simulink model "missile_model"  (R2025a)
settings: Solver=ode4  StartTime=0.0  StopTime=40  FixedStep=0.01  RelTol=1e-5
PreLoadFcn:
  | [aircraft, state] = astDehavillandBeaver();
  | thrustX = getCoefficient(aircraft,"CX","Propeller",Component="Propeller");
model workspace (MATLAB code in the model file + MAT data in the model file):
  inputs0.time = 0
  inputs0.signals(1).dimensions = 1
  inputs0.signals(1).values = -0.104711430294
  inputs0.signals(2).dimensions = 1
  inputs0.signals(2).values = -0.0698725229544
  inputs0.signals(3).dimensions = 1
  inputs0.signals(3).values = -0.000215042330254
  states.time = 0
  states.signals(1).values = 0
  states.signals(1).dimensions = 1
  states.signals(1).label = 'CSTATE'
  states.signals(1).blockName = 'asb6DOFAirframeTemplate/6DOF EOM/6DOF (Euler Angles)/xe,ye,ze'
  states.signals(1).stateName = 'Xe'
  states.signals(1).inReferencedModel = 0
  states.signals(1).sampleTime = [0 0]
  states.signals(2).values = 0
  states.signals(2).dimensions = 1
  states.signals(2).label = 'CSTATE'
  states.signals(2).blockName = 'asb6DOFAirframeTemplate/6DOF EOM/6DOF (Euler Angles)/xe,ye,ze'
  states.signals(2).stateName = 'Ye'
  states.signals(2).inReferencedModel = 0
  states.signals(2).sampleTime = [0 0]
  states.signals(3).values = -2202
  states.signals(3).dimensions = 1
  states.signals(3).label = 'CSTATE'
  states.signals(3).blockName = 'asb6DOFAirframeTemplate/6DOF EOM/6DOF (Euler Angles)/xe,ye,ze'
  states.signals(3).stateName = 'Ze'
  states.signals(3).inReferencedModel = 0
  states.signals(3).sampleTime = [0 0]
  states.signals(4).values = 0.128665353089
  states.signals(4).dimensions = 1
  states.signals(4).label = 'CSTATE'
  states.signals(4).blockName = 'asb6DOFAirframeTemplate/6DOF EOM/6DOF (Euler Angles)/Calculate DCM &
    | Euler Angles/phi
    | theta
    | psi'
  states.signals(4).stateName = 'phi'
  states.signals(4).inReferencedModel = 0
  states.signals(4).sampleTime = [0 0]
  states.signals(5).values = 0.259337659946
  states.signals(5).dimensions = 1
  states.signals(5).label = 'CSTATE'
  states.signals(5).blockName = 'asb6DOFAirframeTemplate/6DOF EOM/6DOF (Euler Angles)/Calculate DCM &
    | Euler Angles/phi
    | theta
    | psi'
  states.signals(5).stateName = 'theta'
  states.signals(5).inReferencedModel = 0
  states.signals(5).sampleTime = [0 0]
  states.signals(6).values = -0.178947917154
  states.signals(6).dimensions = 1
  states.signals(6).label = 'CSTATE'
  states.signals(6).blockName = 'asb6DOFAirframeTemplate/6DOF EOM/6DOF (Euler Angles)/Calculate DCM &
    | Euler Angles/phi
    | theta
    | psi'
  states.signals(6).stateName = 'psi'
  states.signals(6).inReferencedModel = 0
  states.signals(6).sampleTime = [0 0]
  states.signals(7).values = 36.9119692666
  states.signals(7).dimensions = 1
  states.signals(7).label = 'CSTATE'
  states.signals(7).blockName = 'asb6DOFAirframeTemplate/6DOF EOM/6DOF (Euler Angles)/ub,vb,wb'
  states.signals(7).stateName = 'Ubody'
  states.signals(7).inReferencedModel = 0
  states.signals(7).sampleTime = [0 0]
  states.signals(8).values = 8.10720863264
  states.signals(8).dimensions = 1
  states.signals(8).label = 'CSTATE'
  states.signals(8).blockName = 'asb6DOFAirframeTemplate/6DOF EOM/6DOF (Euler Angles)/ub,vb,wb'
  states.signals(8).stateName = 'Vbody'
  states.signals(8).inReferencedModel = 0
  states.signals(8).sampleTime = [0 0]
  states.signals(9).values = 8.82591882596
  states.signals(9).dimensions = 1
  states.signals(9).label = 'CSTATE'
  states.signals(9).blockName = 'asb6DOFAirframeTemplate/6DOF EOM/6DOF (Euler Angles)/ub,vb,wb'
  states.signals(9).stateName = 'Wbody'
  states.signals(9).inReferencedModel = 0
  states.signals(9).sampleTime = [0 0]
  states.signals(10).values = 0
  states.signals(10).dimensions = 1
  states.signals(10).label = 'CSTATE'
  states.signals(10).blockName = 'asb6DOFAirframeTemplate/6DOF EOM/6DOF (Euler Angles)/p,q,r '
  states.signals(10).stateName = 'p'
  states.signals(10).inReferencedModel = 0
  states.signals(10).sampleTime = [0 0]
  states.signals(11).values = 0
  states.signals(11).dimensions = 1
  states.signals(11).label = 'CSTATE'
  states.signals(11).blockName = 'asb6DOFAirframeTemplate/6DOF EOM/6DOF (Euler Angles)/p,q,r '
  states.signals(11).stateName = 'q'
  states.signals(11).inReferencedModel = 0
  states.signals(11).sampleTime = [0 0]
  states.signals(12).values = 0
  states.signals(12).dimensions = 1
  states.signals(12).label = 'CSTATE'
  states.signals(12).blockName = 'asb6DOFAirframeTemplate/6DOF EOM/6DOF (Euler Angles)/p,q,r '
  states.signals(12).stateName = 'r'
  states.signals(12).inReferencedModel = 0
  states.signals(12).sampleTime = [0 0]
  states.signals(13).values = [0 0]
  states.signals(13).dimensions = 2
  states.signals(13).label = 'CSTATE'
  states.signals(13).blockName = 'asb6DOFAirframeTemplate/Environment Model/Dryden Wind Turbulence Model 
    | (Continuous (+q +r))/Filters on velocities/Hwgw(s)/wg_p1'
  states.signals(13).stateName = ''
  states.signals(13).inReferencedModel = 0
  states.signals(13).sampleTime = [0 0]
  states.signals(14).values = [0 0]
  states.signals(14).dimensions = 2
  states.signals(14).label = 'CSTATE'
  states.signals(14).blockName = 'asb6DOFAirframeTemplate/Environment Model/Dryden Wind Turbulence Model 
    | (Continuous (+q +r))/Filters on velocities/Hwgw(s)/wg_p2'
  states.signals(14).stateName = ''
  states.signals(14).inReferencedModel = 0
  states.signals(14).sampleTime = [0 0]
  states.signals(15).values = [0 0]
  states.signals(15).dimensions = 2
  states.signals(15).label = 'CSTATE'
  states.signals(15).blockName = 'asb6DOFAirframeTemplate/Environment Model/Dryden Wind Turbulence Model 
    | (Continuous (+q +r))/Filters on velocities/Hvgw(s)/vg_p1'
  states.signals(15).stateName = ''
  states.signals(15).inReferencedModel = 0
  states.signals(15).sampleTime = [0 0]
  states.signals(16).values = [0 0]
  states.signals(16).dimensions = 2
  states.signals(16).label = 'CSTATE'
  states.signals(16).blockName = 'asb6DOFAirframeTemplate/Environment Model/Dryden Wind Turbulence Model 
    | (Continuous (+q +r))/Filters on velocities/Hvgw(s)/vgw_p2'
  states.signals(16).stateName = ''
  states.signals(16).inReferencedModel = 0
  states.signals(16).sampleTime = [0 0]
  states.signals(17).values = [0 0]
  states.signals(17).dimensions = 2
  states.signals(17).label = 'CSTATE'
  states.signals(17).blockName = 'asb6DOFAirframeTemplate/Environment Model/Dryden Wind Turbulence Model 
    | (Continuous (+q +r))/Filters on velocities/Hugw(s)/ug_p'
  states.signals(17).stateName = ''
  states.signals(17).inReferencedModel = 0
  states.signals(17).sampleTime = [0 0]
  states.signals(18).values = [0 0]
  states.signals(18).dimensions = 2
  states.signals(18).label = 'CSTATE'
  states.signals(18).blockName = 'asb6DOFAirframeTemplate/Environment Model/Dryden Wind Turbulence Model 
    | (Continuous (+q +r))/Filters on angular rates/Hrgw/rgw_p'
  states.signals(18).stateName = ''
  states.signals(18).inReferencedModel = 0
  states.signals(18).sampleTime = [0 0]
  states.signals(19).values = [0 0]
  states.signals(19).dimensions = 2
  states.signals(19).label = 'CSTATE'
  states.signals(19).blockName = 'asb6DOFAirframeTemplate/Environment Model/Dryden Wind Turbulence Model 
    | (Continuous (+q +r))/Filters on angular rates/Hqgw/qgw_p'
  states.signals(19).stateName = ''
  states.signals(19).inReferencedModel = 0
  states.signals(19).sampleTime = [0 0]
  states.signals(20).values = [0 0]
  states.signals(20).dimensions = 2
  states.signals(20).label = 'CSTATE'
  states.signals(20).blockName = 'asb6DOFAirframeTemplate/Environment Model/Dryden Wind Turbulence Model 
    | (Continuous (+q +r))/Filters on angular rates/Hpgw/pgw_p'
  states.signals(20).stateName = ''
  states.signals(20).inReferencedModel = 0
  states.signals(20).sampleTime = [0 0]
  states0.time = 0
  states0.signals(1).values = [0 0 -2202]
  states0.signals(1).dimensions = 3
  states0.signals(1).label = 'CSTATE'
  states0.signals(1).blockName = 'asb6DOFAirframeTemplate/6DOF EOM/6DOF (Euler Angles)/xe,ye,ze'
  states0.signals(1).stateName = ''
  states0.signals(1).inReferencedModel = 0
  states0.signals(1).sampleTime = [0 0]
  states0.signals(2).values = [0.128665353089 0.259337659946 -0.178947917154]
  states0.signals(2).dimensions = 3
  states0.signals(2).label = 'CSTATE'
  states0.signals(2).blockName = 'asb6DOFAirframeTemplate/6DOF EOM/6DOF (Euler Angles)/Calculate DCM &
    | Euler Angles/phi
    | theta
    | psi'
  states0.signals(2).stateName = ''
  states0.signals(2).inReferencedModel = 0
  states0.signals(2).sampleTime = [0 0]
  states0.signals(3).values = [36.9119692666 8.10720863264 8.82591882596]
  states0.signals(3).dimensions = 3
  states0.signals(3).label = 'CSTATE'
  states0.signals(3).blockName = 'asb6DOFAirframeTemplate/6DOF EOM/6DOF (Euler Angles)/ub,vb,wb'
  states0.signals(3).stateName = ''
  states0.signals(3).inReferencedModel = 0
  states0.signals(3).sampleTime = [0 0]
  states0.signals(4).values = [0 0 0]
  states0.signals(4).dimensions = 3
  states0.signals(4).label = 'CSTATE'
  states0.signals(4).blockName = 'asb6DOFAirframeTemplate/6DOF EOM/6DOF (Euler Angles)/p,q,r '
  states0.signals(4).stateName = ''
  states0.signals(4).inReferencedModel = 0
  states0.signals(4).sampleTime = [0 0]
  states0.signals(5).values = [0 0]
  states0.signals(5).dimensions = 2
  states0.signals(5).label = 'CSTATE'
  states0.signals(5).blockName = 'asb6DOFAirframeTemplate/Environment Model/Dryden Wind Turbulence Model 
    | (Continuous (+q +r))/Filters on velocities/Hwgw(s)/wg_p1'
  states0.signals(5).stateName = ''
  states0.signals(5).inReferencedModel = 0
  states0.signals(5).sampleTime = [0 0]
  states0.signals(6).values = [0 0]
  states0.signals(6).dimensions = 2
  states0.signals(6).label = 'CSTATE'
  states0.signals(6).blockName = 'asb6DOFAirframeTemplate/Environment Model/Dryden Wind Turbulence Model 
    | (Continuous (+q +r))/Filters on velocities/Hwgw(s)/wg_p2'
  states0.signals(6).stateName = ''
  states0.signals(6).inReferencedModel = 0
  states0.signals(6).sampleTime = [0 0]
  states0.signals(7).values = [0 0]
  states0.signals(7).dimensions = 2
  states0.signals(7).label = 'CSTATE'
  states0.signals(7).blockName = 'asb6DOFAirframeTemplate/Environment Model/Dryden Wind Turbulence Model 
    | (Continuous (+q +r))/Filters on velocities/Hvgw(s)/vg_p1'
  states0.signals(7).stateName = ''
  states0.signals(7).inReferencedModel = 0
  states0.signals(7).sampleTime = [0 0]
  states0.signals(8).values = [0 0]
  states0.signals(8).dimensions = 2
  states0.signals(8).label = 'CSTATE'
  states0.signals(8).blockName = 'asb6DOFAirframeTemplate/Environment Model/Dryden Wind Turbulence Model 
    | (Continuous (+q +r))/Filters on velocities/Hvgw(s)/vgw_p2'
  states0.signals(8).stateName = ''
  states0.signals(8).inReferencedModel = 0
  states0.signals(8).sampleTime = [0 0]
  states0.signals(9).values = [0 0]
  states0.signals(9).dimensions = 2
  states0.signals(9).label = 'CSTATE'
  states0.signals(9).blockName = 'asb6DOFAirframeTemplate/Environment Model/Dryden Wind Turbulence Model 
    | (Continuous (+q +r))/Filters on velocities/Hugw(s)/ug_p'
  states0.signals(9).stateName = ''
  states0.signals(9).inReferencedModel = 0
  states0.signals(9).sampleTime = [0 0]
  states0.signals(10).values = [0 0]
  states0.signals(10).dimensions = 2
  states0.signals(10).label = 'CSTATE'
  states0.signals(10).blockName = 'asb6DOFAirframeTemplate/Environment Model/Dryden Wind Turbulence Model 
    | (Continuous (+q +r))/Filters on angular rates/Hrgw/rgw_p'
  states0.signals(10).stateName = ''
  states0.signals(10).inReferencedModel = 0
  states0.signals(10).sampleTime = [0 0]
  states0.signals(11).values = [0 0]
  states0.signals(11).dimensions = 2
  states0.signals(11).label = 'CSTATE'
  states0.signals(11).blockName = 'asb6DOFAirframeTemplate/Environment Model/Dryden Wind Turbulence Model 
    | (Continuous (+q +r))/Filters on angular rates/Hqgw/qgw_p'
  states0.signals(11).stateName = ''
  states0.signals(11).inReferencedModel = 0
  states0.signals(11).sampleTime = [0 0]
  states0.signals(12).values = [0 0]
  states0.signals(12).dimensions = 2
  states0.signals(12).label = 'CSTATE'
  states0.signals(12).blockName = 'asb6DOFAirframeTemplate/Environment Model/Dryden Wind Turbulence Model 
    | (Continuous (+q +r))/Filters on angular rates/Hpgw/pgw_p'
  states0.signals(12).stateName = ''
  states0.signals(12).inReferencedModel = 0
  states0.signals(12).sampleTime = [0 0]
  other statements: initialize6DOFSkyHogg;
values from neighbouring files (symbols this model uses):
  Ka = 4.5    [missile.m]
  Kdc = 1.1    [missile.m]
  Ki = 14.3    [missile.m]
  Kr = -0.37    [missile.m]
  l_M0 = 80*d2r    (= 1.3962634016)    [missile.m]
  l_T0 = -2.5*d2r    (= -0.0436332312999)    [missile.m]
  V_T = 900    [missile.m]
  X_M0 = 2000    [missile.m]
  X_T0 = 110    [missile.m]
  Z_M0 = 0    [missile.m]
  Z_T0 = 20000    [missile.m]
libraries: simulink x1
settings Model: Creator=guyle  LastModifiedBy=guyle
settings SolverCC: AlgebraicLoopSolver=TrustRegion  AutoInsertRateTranBlk=on  InsertRTBMode=Never (minimum delay)  MinimalZcImpactIntegration=on  MaxZcPerStep=1.0
settings DataIOCC: ExternalInput=inputs0  InitialState=states  SaveFormat=Array  SaveOutput=off
settings OptimizationCC: EnhancedBackFolding=on  StrengthReduction=on  InitFltsAndDblsToZero=on  DifferentSizesBufferReuse=on
settings DebuggingCC: WriteAfterWriteMsg=DisableAll  AlgebraicLoopMsg=none  FcnCallInpInsideContextMsg=warning  UniqueDataStoreMsg=error  RootOutportRequireBusObject=none  StateNameClashWarn=warning  StrictBusMsg=ErrorOnBusTreatedAsVector  SFUnexpectedBacktrackingDiag=warning  SFNoUnconditionalDefaultTransitionDiag=warning  SFExecutionAtInitializationDiag=none  ArithmeticOperatorsInVariantConditions=warning
settings ModelReferenceCC: EnableRefExpFcnMdlSchedulingChecks=on  PropagateSignalLabelsOutOfModel=off
settings SFSimCC: SimUseLocalCustomCode=off
settings RTWCC: RTWUseLocalCustomCode=off  GPUComputeCapability=3.5  DLArmComputeVersion=19.05
settings CodeAppCC: StateflowObjectComments=on

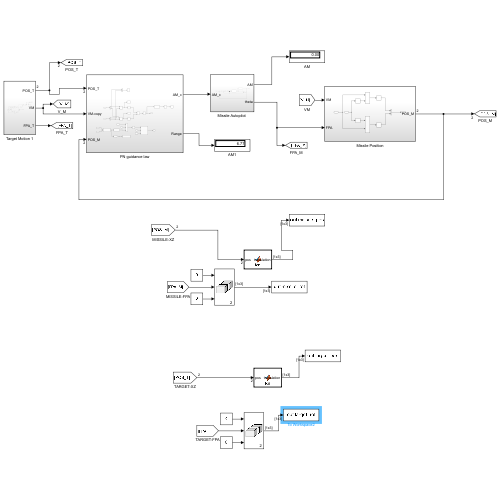
[thumbnail: Simulink's stored preview of the top-level diagram]
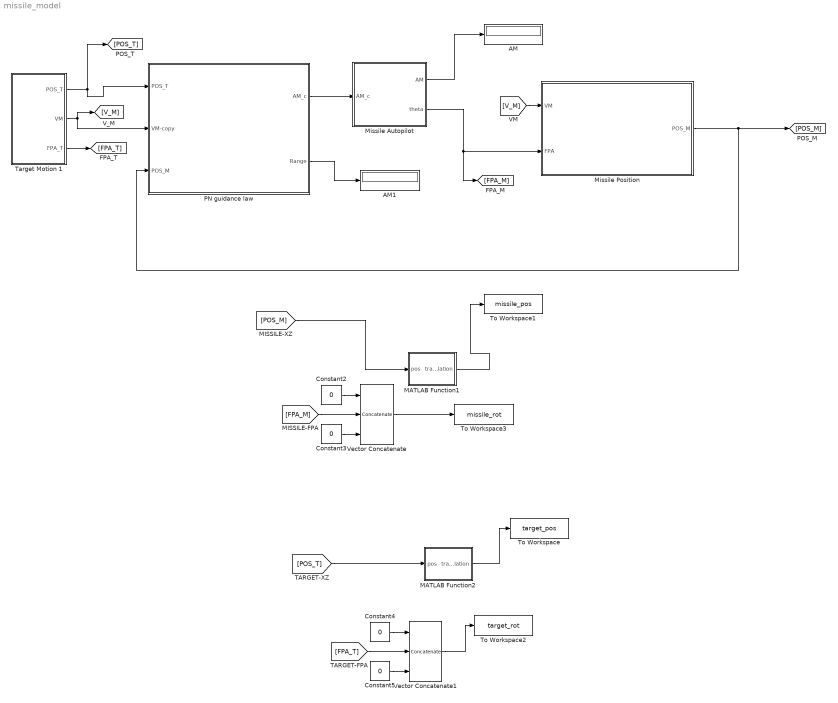
== system missile_model ==
  AM : Display
      settings: Format=bank
  AM1 : Display
      settings: Format=bank
  Constant{2..5} (4 alike) : Constant  Value=0
  MATLAB Function1 : MATLAB Function  TreatAsAtomicUnit=on
  MATLAB Function2 : MATLAB Function  TreatAsAtomicUnit=on
  "Missile Autopilot " : Subsystem
  Missile Position : Subsystem
  PN guidance law : Subsystem
  Target Motion 1 : Subsystem
  To Workspace : ToWorkspace  VariableName=target_pos  SampleTime=.01
      settings: Save2DSignal=2-D array (concatenate along first dimension)
  To Workspace1 : ToWorkspace  VariableName=missile_pos  SampleTime=.01
      settings: Save2DSignal=2-D array (concatenate along first dimension)
  To Workspace2 : ToWorkspace  VariableName=target_rot  SampleTime=.01
      settings: Save2DSignal=2-D array (concatenate along first dimension)
  To Workspace3 : ToWorkspace  VariableName=missile_rot  SampleTime=.01
      settings: Save2DSignal=2-D array (concatenate along first dimension)
  Vector Concatenate : Concatenate  NumInputs=3  Mode=Multidimensional array  ConcatenateDimension=2
  Vector Concatenate1 : Concatenate  NumInputs=3  Mode=Multidimensional array  ConcatenateDimension=2
  wires:
  Target Motion 1/1(POS_T) -> PN guidance law/1(POS_T), [POS_T]
  Target Motion 1/2(VM) -> PN guidance law/2(VM-copy), [V_M]
  [V_M] -> Missile Position/1(VM)
  Missile Position/1(POS_M) -> [POS_M], PN guidance law/3(POS_M)
  PN guidance law/1(AM_c) -> "Missile Autopilot "/1(AM_c)
  "Missile Autopilot "/1(AM) -> AM/1
  "Missile Autopilot "/2(theta) -> Missile Position/2(FPA), [FPA_M]
  PN guidance law/2(Range) -> AM1/1
  Target Motion 1/3(FPA_T) -> [FPA_T]
  [FPA_M] -> Vector Concatenate/2
  Constant2/1 -> Vector Concatenate/1
  Constant3/1 -> Vector Concatenate/3
  Constant4/1 -> Vector Concatenate1/1
  Constant5/1 -> Vector Concatenate1/3
  [FPA_T] -> Vector Concatenate1/2
  Vector Concatenate1/1 -> To Workspace2/1
  Vector Concatenate/1 -> To Workspace3/1
  [POS_M] -> MATLAB Function1/1(pos)
  [POS_T] -> MATLAB Function2/1(pos)
  MATLAB Function2/1(translation) -> To Workspace/1
  MATLAB Function1/1(translation) -> To Workspace1/1

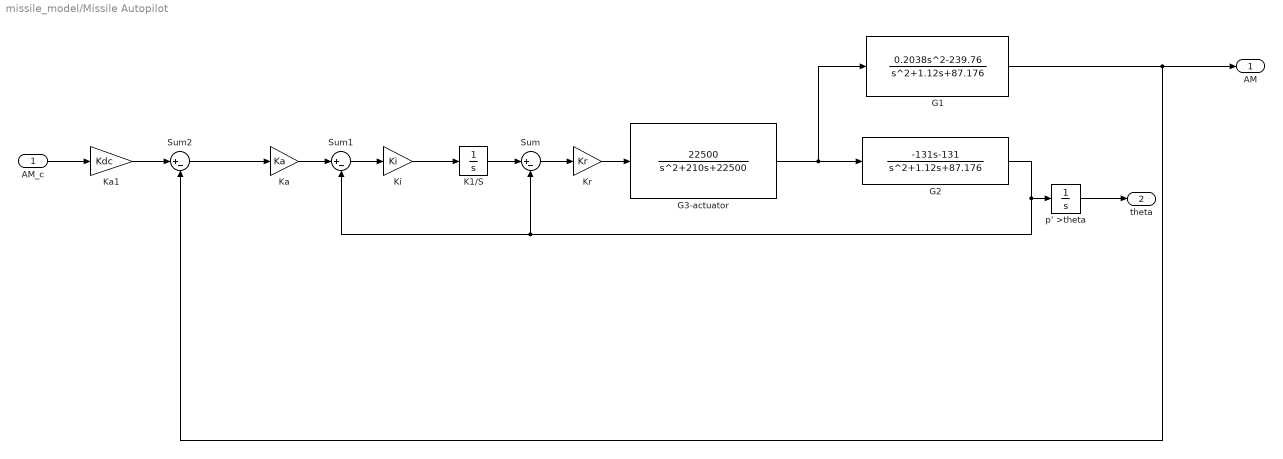
== system missile_model/Missile Autopilot  ==
  AM_c : Inport
  G1 : TransferFcn  Numerator=[0.2038 0 -239.76]  Denominator=[1 1.12 87.176]
  G2 : TransferFcn  Numerator=[-131 -131]  Denominator=[1 1.12 87.176]
  "G3-actuator " : TransferFcn  Numerator=[22500]  Denominator=[1 210 22500]
  K1/S : Integrator
  Ka : Gain  Gain=Ka
  Ka1 : Gain  Gain=Kdc
  Ki : Gain  Gain=Ki
  Kr : Gain  Gain=Kr
  Sum : Sum  Inputs=|+-
  Sum1 : Sum  Inputs=|+-
  Sum2 : Sum  Inputs=|+-
  p' >theta : Integrator  InitialCondition=l_M0
  AM : Outport
  theta : Outport  Port=2
  wires:
  G1/1 -> AM/1, Sum2/2
  G2/1 -> p' >theta/1, Sum1/2, Sum/2
  Sum/1 -> Kr/1
  Ki/1 -> K1/S/1
  Ka/1 -> Sum1/1
  Sum1/1 -> Ki/1
  "G3-actuator "/1 -> G1/1, G2/1
  Ka1/1 -> Sum2/1
  Sum2/1 -> Ka/1
  AM_c/1 -> Ka1/1
  Kr/1 -> "G3-actuator "/1
  p' >theta/1 -> theta/1
  K1/S/1 -> Sum/1

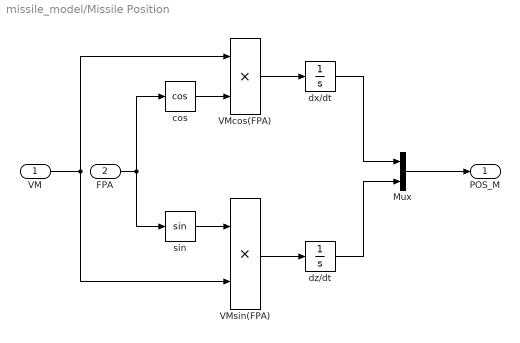
== system missile_model/Missile Position ==
  VM : Inport
  FPA : Inport  Port=2
  Mux : Mux  Inputs=2
  VMcos(FPA) : Product
  VMsin(FPA) : Product
  cos : Trigonometry  Operator=cos
  dx/dt : Integrator  InitialCondition=X_M0
  dz/dt : Integrator  InitialCondition=Z_M0
  sin : Trigonometry
  POS_M : Outport
  wires:
  VMsin(FPA)/1 -> dz/dt/1
  dz/dt/1 -> Mux/2
  sin/1 -> VMsin(FPA)/1
  dx/dt/1 -> Mux/1
  VMcos(FPA)/1 -> dx/dt/1
  FPA/1 -> sin/1, cos/1
  Mux/1 -> POS_M/1
  VM/1 -> VMsin(FPA)/2, VMcos(FPA)/1
  cos/1 -> VMcos(FPA)/2

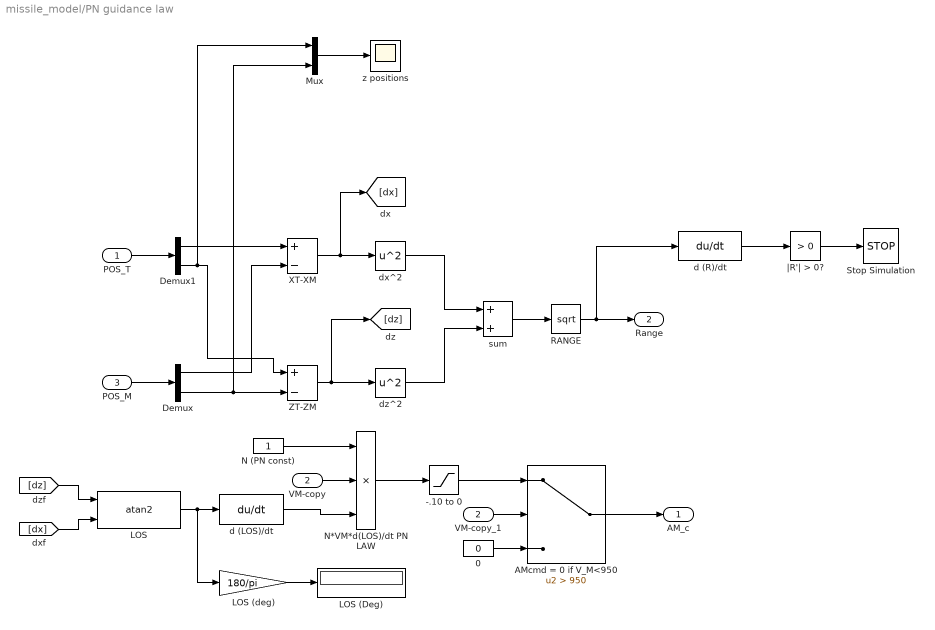
== system missile_model/PN guidance law ==
  POS_T : Inport
  VM-copy : Inport  Port=2
  POS_M : Inport  Port=3
  -.10 to 0 : Saturate  UpperLimit=0  LowerLimit=-0.1
  0 : Constant  Value=0
  "AMcmd = 0 if V_M<950 " : Switch  Criteria=u2 > Threshold  Threshold=950  SaturateOnIntegerOverflow=off  InputSameDT=off
  Demux : Demux  Outputs=2
  Demux1 : Demux  Outputs=2
  LOS : Trigonometry  Operator=atan2
  LOS (Deg) : Display
  LOS (deg) : Gain  Gain=180/pi
  Mux : Mux  Inputs=2
  N (PN const) : Constant
  N*VM*d(LOS)/dt PN LAW : Product  Inputs=3
  "RANGE " : Sqrt
  Stop Simulation : Stop
  VM-copy_1 : InportShadow  Port=2
  XT-XM : Sum  Inputs=+-
  ZT-ZM : Sum  Inputs=+-
  d (LOS)/dt : Derivative
  d (R)/dt : Derivative
  dx^2 : Math  Operator=square
  dz^2 : Math  Operator=square
  sum : Sum
  "z positions " : Scope
      settings: ActiveDisplayYMinimum=0  ActiveDisplayYMaximum=20000
  |R'| > 0? : simulink/Logic and Bit Operations/Compare To Zero  relop=>  OutDataTypeStr=boolean
  AM_c : Outport
  Range : Outport  Port=2
  wires:
  XT-XM/1 -> [dx], dx^2/1
  "AMcmd = 0 if V_M<950 "/1 -> AM_c/1
  LOS/1 -> LOS (deg)/1, d (LOS)/dt/1
  dx^2/1 -> sum/1
  VM-copy_1/1 -> "AMcmd = 0 if V_M<950 "/2
  sum/1 -> "RANGE "/1
  d (LOS)/dt/1 -> N*VM*d(LOS)/dt PN LAW/3
  Demux/1 -> XT-XM/2
  Demux1/1 -> XT-XM/1
  Demux/2 -> Mux/2, ZT-ZM/2
  Demux1/2 -> Mux/1, ZT-ZM/1
  "RANGE "/1 -> Range/1, d (R)/dt/1
  POS_M/1 -> Demux/1
  POS_T/1 -> Demux1/1
  LOS (deg)/1 -> LOS (Deg)/1
  [dz] -> LOS/1
  Mux/1 -> "z positions "/1
  dz^2/1 -> sum/2
  VM-copy/1 -> N*VM*d(LOS)/dt PN LAW/2
  ZT-ZM/1 -> [dz], dz^2/1
  0/1 -> "AMcmd = 0 if V_M<950 "/3
  -.10 to 0/1 -> "AMcmd = 0 if V_M<950 "/1
  [dx] -> LOS/2
  d (R)/dt/1 -> |R'| > 0?/1
  N (PN const)/1 -> N*VM*d(LOS)/dt PN LAW/1
  N*VM*d(LOS)/dt PN LAW/1 -> -.10 to 0/1
  |R'| > 0?/1 -> Stop Simulation/1

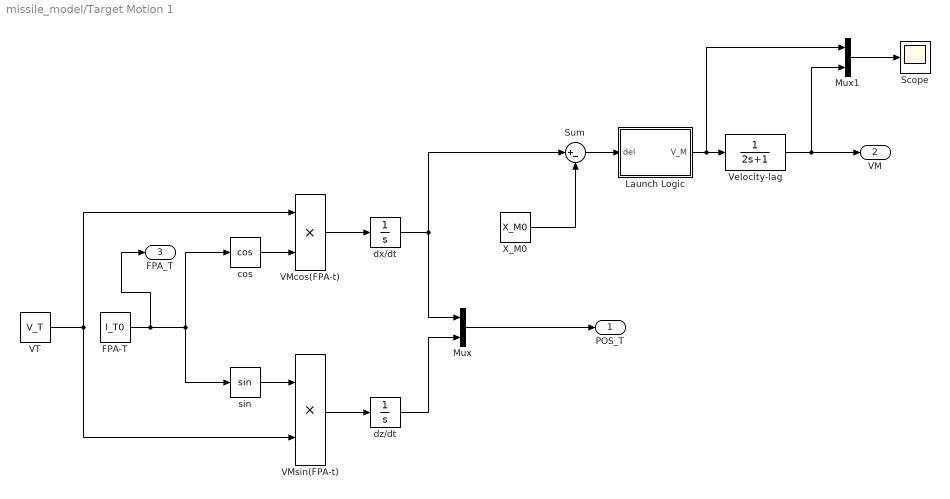
== system missile_model/Target Motion 1 ==
  FPA-T : Constant  Value=l_T0
  "Launch Logic " : MATLAB Function  TreatAsAtomicUnit=on
  Mux : Mux  Inputs=2
  Mux1 : Mux  Inputs=2
  Scope : Scope
  Sum : Sum  Inputs=|+-
  VMcos(FPA-t) : Product
  VMsin(FPA-t) : Product
  VT : Constant  Value=V_T
  Velocity-lag : TransferFcn  Denominator=[2 1]
  X_M0 : Constant  Value=X_M0
  cos : Trigonometry  Operator=cos
  dx/dt : Integrator  InitialCondition=X_T0
  dz/dt : Integrator  InitialCondition=Z_T0
  sin : Trigonometry
  POS_T : Outport
  VM : Outport  Port=2
  FPA_T : Outport  Port=3
  wires:
  X_M0/1 -> Sum/2
  Sum/1 -> "Launch Logic "/1(del)
  Mux/1 -> POS_T/1
  VT/1 -> VMsin(FPA-t)/2, VMcos(FPA-t)/1
  "Launch Logic "/1(V_M) -> Velocity-lag/1, Mux1/1
  cos/1 -> VMcos(FPA-t)/2
  dx/dt/1 -> Sum/1, Mux/1
  dz/dt/1 -> Mux/2
  VMsin(FPA-t)/1 -> dz/dt/1
  Mux1/1 -> Scope/1
  Velocity-lag/1 -> Mux1/2, VM/1
  FPA-T/1 -> FPA_T/1, cos/1, sin/1
  sin/1 -> VMsin(FPA-t)/1
  VMcos(FPA-t)/1 -> dx/dt/1

== matlab function missile_model/MATLAB Function2 ==
  data: pos input; translation output
function translation = fcn(pos)
    % pos is [x, z] (1x2 vector)
    % Output: [x, 0, z] (1x3 vector)
    
    translation = [pos(1), 0, pos(2)];
end

== matlab function missile_model/MATLAB Function1 ==
  data: pos input; translation output
function translation = fcn(pos)
    % pos is [x, z] (1x2 vector)
    % Output: [x, 0, z] (1x3 vector)
    
    translation = [pos(1), 0, pos(2)];
end

== matlab function missile_model/Target Motion 1/Launch Logic  ==
  settings: updateMethod=DISCRETE
  data: del input; V_M output
function V_M = fcn(del)


persistent f
persistent Vel

if isempty(f)
    f = 0;
end 
if isempty(Vel)
    Vel=0;
end 

if f == 0 && del > -200
    f = 1;
    Vel = 1021; %missile speed
end



V_M = Vel;
